simulink model "rigidbodyB"  (Simulink 6.1)
settings: Solver=ode45  StartTime=0.0  StopTime=10.0  RelTol=1e-3
libraries: simulink x1
settings Model: LastModifiedBy=okawa
settings DebuggingCC: SolverPrmCheckMsg=warning

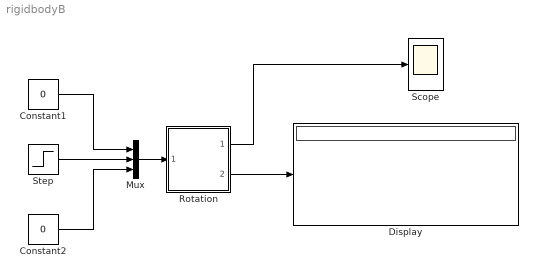
== system rigidbodyB ==
  Constant1 : Constant  Value=0
  Constant2 : Constant  Value=0
  Display : Display
  Mux : Mux  Inputs=3
  Rotation : Subsystem
  Scope : Scope
  Step : Step  SampleTime=0
  wires:
  Constant1/1 -> Mux/1
  Step/1 -> Mux/2
  Constant2/1 -> Mux/3
  Mux/1 -> Rotation/1(Torque)
  Rotation/1(Omega) -> Scope/1
  Rotation/2(Theta) -> Display/1

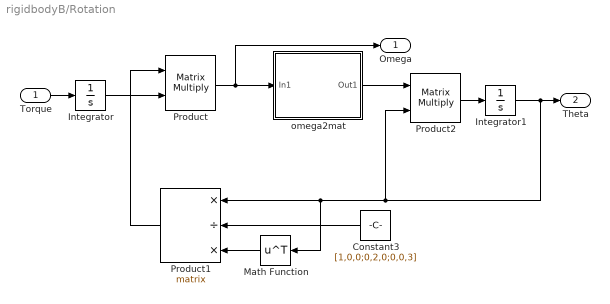
== system rigidbodyB/Rotation ==
  Torque : Inport  Port=1  LatchInput=off
  Constant3 : Constant  Orientation=left  Value=[1,0,0;0,2,0;0,0,3]  VectorParams1D=off
  Integrator : Integrator
  Integrator1 : Integrator  InitialCondition=[1,0,0;0,1,0;0,0,1]
  Math Function : Math  Orientation=left  Operator=transpose  SaturateOnIntegerOverflow=on
  Product : Product  Inputs=**  Multiplication=Matrix(*)  RndMeth=Zero
  Product1 : Product  Orientation=left  Inputs=*/*  Multiplication=Matrix(*)  RndMeth=Zero
  Product2 : Product  Inputs=**  Multiplication=Matrix(*)  RndMeth=Zero
  omega2mat : Subsystem
  Omega : Outport
  Theta : Outport  Port=2
  wires:
  Integrator/1 -> Product/2
  Product/1 -> Omega/1, omega2mat/1(In1)
  omega2mat/1(Out1) -> Product2/1
  Product2/1 -> Integrator1/1
  Integrator1/1 -> Product1/1, Math Function/1, Product2/2, Theta/1
  Constant3/1 -> Product1/2
  Math Function/1 -> Product1/3
  Product1/1 -> Product/1
  Torque/1 -> Integrator/1

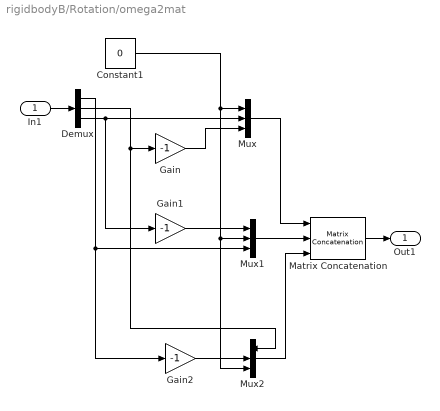
== system rigidbodyB/Rotation/omega2mat ==
  In1 : Inport  Port=1  LatchInput=off
  Constant1 : Constant  Value=0
  Demux : Demux  Outputs=3
  Gain : Gain  Gain=-1
  Gain1 : Gain  Gain=-1
  Gain2 : Gain  Gain=-1
  Matrix Concatenation : simulink/Math Operations/Matrix Concatenation  numInports=3  catMethod=Horizontal
  Mux : Mux  Inputs=3
  Mux1 : Mux  Inputs=3
  Mux2 : Mux  Inputs=3
  Out1 : Outport
  wires:
  Constant1/1 -> Mux/1, Mux1/2, Mux2/3
  Demux/2 -> Gain/1, Mux2/1
  Gain/1 -> Mux/3
  Demux/3 -> Mux/2, Gain1/1
  Gain1/1 -> Mux1/1
  Demux/1 -> Mux1/3, Gain2/1
  Gain2/1 -> Mux2/2
  Mux/1 -> Matrix Concatenation/1
  Mux1/1 -> Matrix Concatenation/2
  Mux2/1 -> Matrix Concatenation/3
  In1/1 -> Demux/1
  Matrix Concatenation/1 -> Out1/1
